simulink model "PX32s"  (R2015b)
settings: Solver=VariableStepAuto  StartTime=0.0  StopTime=10.0  RelTol=1e-3
settings Model: Creator=xmax1946  LastModifiedBy=xmax1946

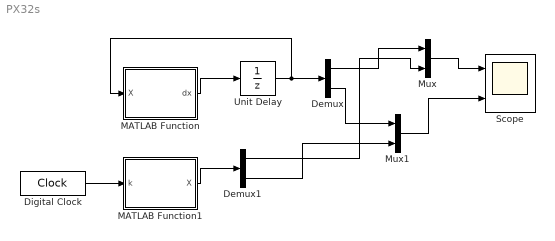
== system PX32s ==
  Demux : Demux  Outputs=2
  Demux1 : Demux  Outputs=2
  Digital Clock : DigitalClock
  MATLAB Function : MATLAB Function  TreatAsAtomicUnit=on
  MATLAB Function1 : MATLAB Function  TreatAsAtomicUnit=on
  Mux : Mux  Inputs=2
  Mux1 : Mux  Inputs=2
  Scope : Scope  NumInputPorts=2
  Unit Delay : UnitDelay  InitialCondition=[-1;4]  SampleTime=-1
  wires:
  MATLAB Function/1(dx) -> Unit Delay/1
  Unit Delay/1 -> Demux/1, MATLAB Function/1(X)
  Digital Clock/1 -> MATLAB Function1/1(k)
  Mux/1 -> Scope/1
  Mux1/1 -> Scope/2
  Demux/1 -> Mux/1
  MATLAB Function1/1(X) -> Demux1/1
  Demux1/1 -> Mux/2
  Demux/2 -> Mux1/1
  Demux1/2 -> Mux1/2

== matlab function PX32s/MATLAB Function1 ==
  data: X output; k input
function X  = fcn(k)

X=[ (85*(-2/5)^k)/63 - (52*(1/2)^k)/9 + 24/7
 52/7 - (34*(-2/5)^k)/63 - (26*(1/2)^k)/9];

== matlab function PX32s/MATLAB Function ==
  data: dx output; X input
function dx = fcn(X)
A=[0,1;.2,.1];
B=[.4;-.6];

dx=A*X+B*(-10);
